simulink model "Project4_Trial"  (R2024b)
settings: Solver=VariableStepAuto  StartTime=0.0  StopTime=10.0  RelTol=1e-3
values from neighbouring files (symbols this model uses):
  b = 0.1    [Project4_run.m]
  F = 10    [Project4_run.m]
  k = 10    [Project4_run.m]
  M = 1    [Project4_run.m]
settings Model: Creator=szala  LastModifiedBy=szala

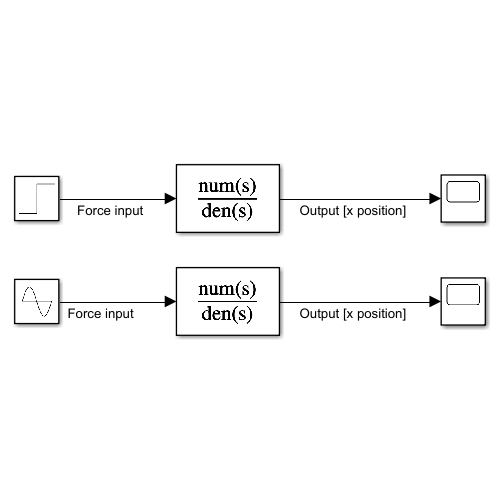
[thumbnail: Simulink's stored preview of the top-level diagram]
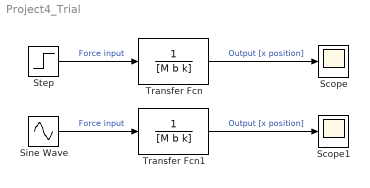
== system Project4_Trial ==
  Scope : Scope
  Scope1 : Scope
  Sine Wave : Sin  SampleTime=0
  Step : Step  After=F  SampleTime=0
  Transfer Fcn : TransferFcn  Denominator=[M b k]
  Transfer Fcn1 : TransferFcn  Denominator=[M b k]
  wires:
  Step/1 -> Transfer Fcn/1  "Force input"
  Transfer Fcn/1 -> Scope/1  "Output [x position]"
  Transfer Fcn1/1 -> Scope1/1  "Output [x position]"
  Sine Wave/1 -> Transfer Fcn1/1  "Force input"
